simulink model "Lab3_zad2"  (Simulink 7.4)
settings: Solver=ode3  StartTime=0.0  StopTime=5.0  FixedStep=0.001  RelTol=1e-3
values from neighbouring files (symbols this model uses):
  m1 = [1 1 0 0]    [Lab2_zad3.m]    (also in Lab2_zad4.m; Lab2_zad5.m; Lab2_zad6.m; Lab4_zad6.m = abs(y1))
  m2 = [ 0 0 1 1 0 0]    [Lab2_zad3.m]    (also in Lab2_zad4.m; Lab4_zad6.m = abs(y2))
undefined symbols (not defined in the file or in its folder): c1, c2, k1, k2
settings Model: Creator=Tomek  LastModifiedBy=Tomek

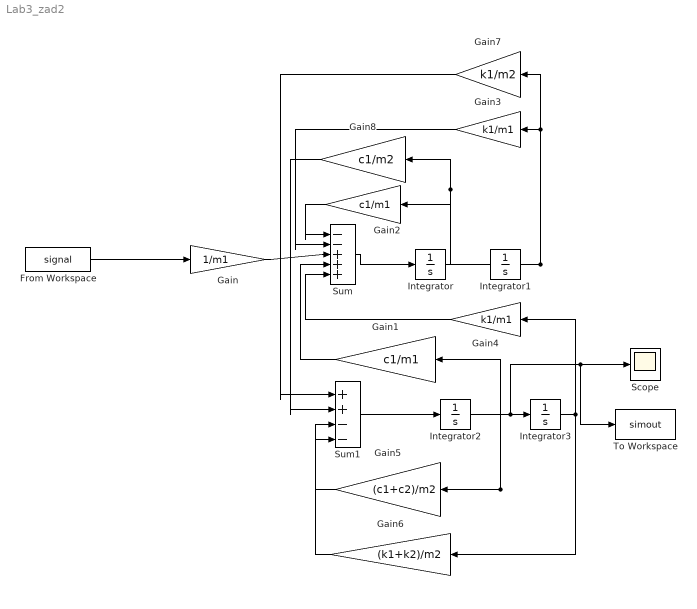
== system Lab3_zad2 ==
  From Workspace : FromWorkspace  VariableName=signal  SampleTime=0
  Gain : Gain  Gain=1/m1  ParameterDataType=fixdt(1, 16)  ParameterScaling=2^0  OutDataType=fixdt(1, 16)  OutScaling=2^0
  Gain1 : Gain  Gain=c1/m1  ParameterDataType=fixdt(1, 16)  ParameterScaling=2^0  OutDataType=fixdt(1, 16)  OutScaling=2^0
  Gain2 : Gain  Gain=c1/m1  ParameterDataType=fixdt(1, 16)  ParameterScaling=2^0  OutDataType=fixdt(1, 16)  OutScaling=2^0
  Gain3 : Gain  Gain=k1/m1  ParameterDataType=fixdt(1, 16)  ParameterScaling=2^0  OutDataType=fixdt(1, 16)  OutScaling=2^0
  Gain4 : Gain  Gain=k1/m1  ParameterDataType=fixdt(1, 16)  ParameterScaling=2^0  OutDataType=fixdt(1, 16)  OutScaling=2^0
  Gain5 : Gain  Gain=(c1+c2)/m2  ParameterDataType=fixdt(1, 16)  ParameterScaling=2^0  OutDataType=fixdt(1, 16)  OutScaling=2^0
  Gain6 : Gain  Gain=(k1+k2)/m2  ParameterDataType=fixdt(1, 16)  ParameterScaling=2^0  OutDataType=fixdt(1, 16)  OutScaling=2^0
  Gain7 : Gain  Gain=k1/m2  ParameterDataType=fixdt(1, 16)  ParameterScaling=2^0  OutDataType=fixdt(1, 16)  OutScaling=2^0
  Gain8 : Gain  Gain=c1/m2  ParameterDataType=fixdt(1, 16)  ParameterScaling=2^0  OutDataType=fixdt(1, 16)  OutScaling=2^0
  Integrator{,1..3} (4 alike) : Integrator
  Scope : Scope
      settings: TimeRange=5  YMin=-6.532375731695502e+129  YMax=-1.353278090507885e+129
  Sum : Sum  Inputs=|--+++  OutDataType=fixdt(1, 16)  OutScaling=2^0
  Sum1 : Sum  Inputs=|++--  OutDataType=fixdt(1, 16)  OutScaling=2^0
  To Workspace : ToWorkspace  VariableName=simout  SampleTime=-1  SaveFormat=Structure
  wires:
  Sum/1 -> Integrator/1
  Integrator/1 -> Integrator1/1, Gain2/1, Gain8/1
  Sum1/1 -> Integrator2/1
  Integrator2/1 -> Gain1/1, Gain5/1, Integrator3/1, Scope/1, To Workspace/1
  Gain/1 -> Sum/3
  Gain2/1 -> Sum/1
  Integrator1/1 -> Gain3/1, Gain7/1
  Gain3/1 -> Sum/2
  Integrator3/1 -> Gain6/1, Gain4/1
  Gain1/1 -> Sum/4
  Gain4/1 -> Sum/5
  Gain5/1 -> Sum1/4
  Gain6/1 -> Sum1/3
  Gain7/1 -> Sum1/1
  Gain8/1 -> Sum1/2
  From Workspace/1 -> Gain/1
